simulink model "signali"  (R2018a)
settings: Solver=ode4  StartTime=0.0  StopTime=100  RelTol=1e-3
undefined symbols (not defined in the file or in its folder): i
libraries: simulink x1
settings Model: Creator=Teodor  LastModifiedBy=Teodor

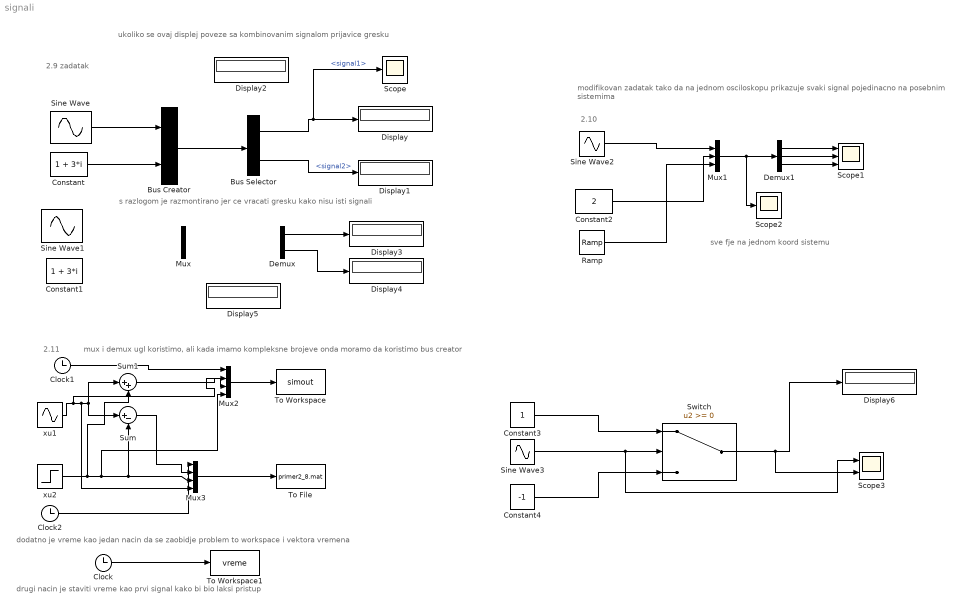
== system signali ==
  note: drugi nacin je staviti vreme kao prvi signal kako bi bio laksi pristup
  note: mux i demux ugl koristimo, ali kada imamo kompleksne brojeve onda moramo da koristimo bus creator
  note: dodatno je vreme kao jedan nacin da se zaobidje problem to workspace i vektora vremena
  note: sve fje na jednom koord sistemu
  note: modifikovan zadatak tako da na jednom osciloskopu prikazuje svaki signal pojedinacno na posebnim sistemima
  note: ukoliko se ovaj displej poveze sa kombinovanim signalom prijavice gresku
  note: s razlogom je razmontirano jer ce vracati gresku kako nisu isti signali
  note: 2.11
  note: 2.10
  note: 2.9 zadatak
  Bus Creator : BusCreator  Inputs=2
  Bus Selector : BusSelector  OutputSignals=signal1,signal2
  Clock : Clock
  Clock1 : Clock
  Clock2 : Clock
  Constant : Constant  Value=1 + 3*i
  Constant1 : Constant  Value=1 + 3*i
  Constant2 : Constant  Value=2
  Constant3 : Constant
  Constant4 : Constant  Value=-1
  Demux : Demux  Outputs=2
  Demux1 : Demux  Outputs=3
  Display{,1..6} (7 alike) : Display
  Mux : Mux  Inputs=2
  Mux1 : Mux  Inputs=3
  Mux2 : Mux
  Mux3 : Mux
  Ramp : simulink/Sources/Ramp  slope=0.5  start=0  InitialOutput=0
  Scope : Scope
  Scope1 : Scope  NumInputPorts=3
  Scope2 : Scope
  Scope3 : Scope  NumInputPorts=2
  Sine Wave : Sin  Amplitude=2  Frequency=3  Phase=pi/4  SampleTime=0
  Sine Wave1 : Sin  Amplitude=2  Frequency=3  Phase=pi/4  SampleTime=0
  Sine Wave2 : Sin  Phase=pi/2  SampleTime=0
  Sine Wave3 : Sin  Frequency=0.5  SampleTime=0
  Sum : Sum  Inputs=|+-
  Sum1 : Sum  Inputs=|++
  Switch : Switch
  To File : ToFile  Filename=primer2_8.mat  MatrixName=izlaz
  To Workspace : ToWorkspace  VariableName=simout  SampleTime=-1
  To Workspace1 : ToWorkspace  VariableName=vreme  SampleTime=-1
  "xu1 " : Sin  SampleTime=0
  "xu2 " : Step  After=2  SampleTime=0
  wires:
  Sine Wave/1 -> Bus Creator/1
  Constant/1 -> Bus Creator/2
  Bus Creator/1 -> Bus Selector/1
  Bus Selector/1 -> Scope/1, Display/1  "<signal1>"
  Bus Selector/2 -> Display1/1  "<signal2>"
  Demux/1 -> Display3/1
  Demux/2 -> Display4/1
  Constant2/1 -> Mux1/2
  Ramp/1 -> Mux1/3
  Sine Wave2/1 -> Mux1/1
  Mux1/1 -> Scope2/1, Demux1/1
  Demux1/1 -> Scope1/1
  Demux1/2 -> Scope1/2
  Demux1/3 -> Scope1/3
  "xu1 "/1 -> Mux2/2, Mux3/4, Sum/1, Sum1/1
  "xu2 "/1 -> Mux2/4, Mux3/3, Sum/2, Sum1/2
  Sum1/1 -> Mux2/3
  Mux2/1 -> To Workspace/1
  Sum/1 -> Mux3/2
  Mux3/1 -> To File/1
  Clock/1 -> To Workspace1/1
  Clock1/1 -> Mux2/1
  Clock2/1 -> Mux3/1
  Constant4/1 -> Switch/3
  Constant3/1 -> Switch/1
  Sine Wave3/1 -> Scope3/1, Switch/2
  Switch/1 -> Scope3/2, Display6/1
